simulink model "system_control"  (R2025b)
settings: Solver=VariableStepAuto  StartTime=0.0  StopTime=1  RelTol=1e-3
values from neighbouring files (symbols this model uses):
  adc_gain = (lim_adc(2)+1)/lim_voltage(2)    [sys_control.m]
  c1 = polyfit(lim_angles, lim_voltage, 1)    [sys_control.m]
  c2 = polyfit(lim_adc, lim_robot_speed, 1)    [sys_control.m]
  c3 = polyfit(lim_adc, lim_robot_angular_velocity, 1)    [sys_control.m]
  c4 = polyfit([0, lim_motor_speed(2)], lim_pwm, 1)    [sys_control.m]
  den_motor_tf = [J*La, J*Ra+b*La, b*Ra+Kt^2]    [sys_control.m]
  forward_kinematics = [ ... (first row only)    [sys_control.m]
  gear_ratio = 1/190    (= 0.00526315789474)    [sys_control.m]
  inverse_kinematics = [ ... (first row only)    [sys_control.m]
  lim_adc = [0, 2^bits-1]    [sys_control.m]
  lim_pwm = [0, 1]    [sys_control.m]
  lim_robot_angular_velocity = [-kinematic_resp(2), kinematic_resp(2)]    [sys_control.m]
  lim_robot_speed = [-kinematic_resp(1), kinematic_resp(1)]    [sys_control.m]
  lim_voltage = [0, 5]    [sys_control.m]
  noise_bias = 0    [sys_control.m]
  noise_bias_2 = 0    [sys_control.m]
  noise_frequency = 1000    [sys_control.m]
  noise_frequency_2 = 10000    [sys_control.m]
  noise_gain = 0.001    [sys_control.m]
  noise_gain_2 = 0.01    [sys_control.m]
  num_motor_tf = Kt    (= 0.076)    [sys_control.m]
  R = 0.3    [sys_control.m]
  vin = 24    [sys_control.m]
libraries: dspstat3 x2, simulink x2, dspfdesign x2, simulink_extras x1

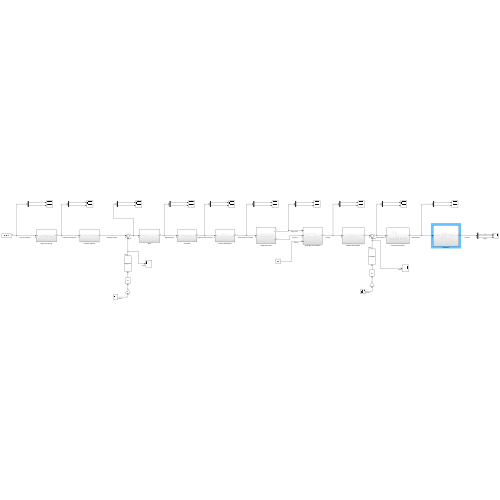
[thumbnail: Simulink's stored preview of the top-level diagram]
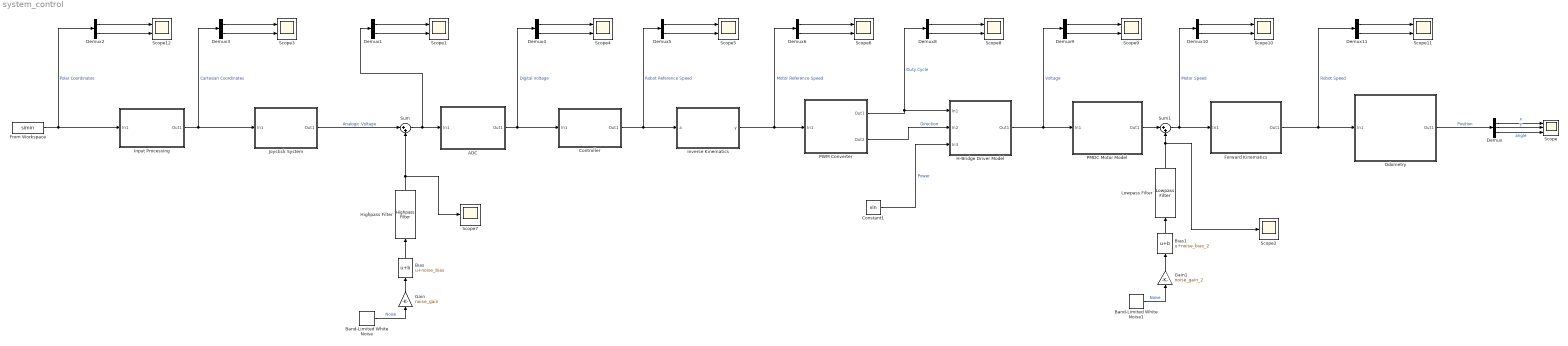
== system system_control ==
  ADC : Subsystem
  Band-Limited White Noise : simulink/Sources/Band-Limited White Noise  Cov=noise_power  Ts=1/noise_frequency  seed=[23341]
  Band-Limited White Noise1 : simulink/Sources/Band-Limited White Noise  Cov=noise_power_2  Ts=1/noise_frequency_2  seed=[23341]
  Bias : Bias  Bias=noise_bias  SaturateOnIntegerOverflow=off
  Bias1 : Bias  Bias=noise_bias_2  SaturateOnIntegerOverflow=off
  Constant1 : Constant  Value=vin
  Controller : Subsystem
  Demux : Demux  Outputs=3
  Demux{1..6,8..11} (10 alike) : Demux  Outputs=2
  Forward Kinematics : Subsystem
  From Workspace : FromWorkspace  VariableName=simin  OutputAfterFinalValue=Holding final value
  Gain : Gain  Gain=noise_gain
  Gain1 : Gain  Gain=noise_gain_2
  H-Bridge Driver Model : Subsystem
  Highpass Filter : dspfdesign/Highpass Filter  FilterType=FIR  DesignForMinimumOrder=on  FilterOrder=50  StopbandFrequency=10  PassbandFrequency=400  StopbandAttenuation=80  PassbandRipple=0.1  SampleRateMode=Specify on dialog  SampleRate=10000  SimulateUsing=Interpreted execution  roundingMode=Floor  coeffsDataTypeStr=fixdt(1,16)
  Input Processing : Subsystem
  Inverse Kinematics : Subsystem
  Joystick System : Subsystem
  Lowpass Filter : dspfdesign/Lowpass Filter  FilterType=FIR  DesignForMinimumOrder=on  FilterOrder=50  PassbandFrequency=8  StopbandFrequency=15  PassbandRipple=0.1  StopbandAttenuation=80  SampleRateMode=Specify on dialog  SampleRate=1000  SimulateUsing=Interpreted execution  roundingMode=Floor  coeffsDataTypeStr=fixdt(1,16)
  Odometry : Subsystem
  PMDC Motor Model : Subsystem
  PWM Converter : Subsystem
  Scope : Scope  NumInputPorts=3
      settings: ActiveDisplayYMinimum=-0.038312008816217151  ActiveDisplayYMaximum=0.34315381688886831  DataLoggingVariableName=odometry  DataLoggingSaveFormat=Structure
  Scope{1,3..6,8..12} (10 alike) : Scope  NumInputPorts=2
      Scope1 settings: ActiveDisplayYMinimum=1.060489809937327  ActiveDisplayYMaximum=5.7930389193730329  DataLoggingVariableName=joystick_analogic_voltage  DataLoggingSaveFormat=Structure
      Scope10 settings: ActiveDisplayYMinimum=-0.22999768707174573  ActiveDisplayYMaximum=0.57575148791845487  DataLoggingVariableName=motor_speed_rbv  DataLoggingSaveFormat=Structure
      Scope11 settings: ActiveDisplayYMinimum=-0.016441629327696137  ActiveDisplayYMaximum=0.1239488307824286  DataLoggingVariableName=robot_speed_rbv  DataLoggingSaveFormat=Structure
      Scope12 settings: ActiveDisplayYMinimum=-0.4195243112740431  ActiveDisplayYMaximum=1.1577249234748936  DataLoggingVariableName=input  DataLoggingSaveFormat=Structure
      Scope3 settings: ActiveDisplayYMinimum=-0.19779285643508393  ActiveDisplayYMaximum=1.1330880951594537  DataLoggingVariableName=joystick_inp  DataLoggingSaveFormat=Structure
      Scope4 settings: ActiveDisplayYMinimum=11.349880751221576  ActiveDisplayYMaximum=1081.1380282237869  DataLoggingVariableName=adc  DataLoggingSaveFormat=Structure
      Scope5 settings: ActiveDisplayYMinimum=0.074969930142674279  ActiveDisplayYMaximum=0.0752153728208186  DataLoggingVariableName=robot_speed_reference  DataLoggingSaveFormat=Structure
      Scope6 settings: ActiveDisplayYMinimum=-0.86358361035381748  ActiveDisplayYMaximum=0.54521612594059543  DataLoggingVariableName=motor_speed_reference  DataLoggingSaveFormat=Structure
      Scope8 settings: ActiveDisplayYMinimum=-0.12499999999999997  ActiveDisplayYMaximum=1.125  DataLoggingVariableName=pwm_duty_cycle  DataLoggingSaveFormat=Structure
      Scope9 settings: ActiveDisplayYMinimum=-29.510263929618766  ActiveDisplayYMaximum=25.592375366568909  DataLoggingVariableName=h_bridge_voltage  DataLoggingSaveFormat=Structure
  Scope2 : Scope
      settings: ActiveDisplayYMinimum=-0.30863024342846962  ActiveDisplayYMaximum=0.11012899050092259  DataLoggingVariableName=motor_speed_rbv1  DataLoggingSaveFormat=Structure
  Scope7 : Scope
      settings: ActiveDisplayYMinimum=-0.92976317089904748  ActiveDisplayYMaximum=0.28796558033489961  DataLoggingVariableName=motor_speed_rbv2  DataLoggingSaveFormat=Structure
  Sum : Sum  Inputs=|++
  Sum1 : Sum  Inputs=|++
  wires:
  Controller/1(Out1) -> Demux5/1, Inverse Kinematics/1(a)  "Robot Reference Speed"
  Inverse Kinematics/1(y) -> Demux6/1, PWM Converter/1(In1)  "Motor Reference Speed"
  PWM Converter/1(Out1) -> H-Bridge Driver Model/1(In1), Demux8/1  "Duty Cycle"
  H-Bridge Driver Model/1(Out1) -> Demux9/1, PMDC Motor Model/1(In1)  "Voltage"
  PMDC Motor Model/1(Out1) -> Sum1/1
  Demux1/2 -> Scope1/2
  Joystick System/1(Out1) -> Sum/1  "Analogic Voltage"
  Demux1/1 -> Scope1/1
  Sum/1 -> Demux1/1, ADC/1(In1)
  Band-Limited White Noise/1 -> Gain/1  "Noise"
  Bias/1 -> Highpass Filter/1
  Gain/1 -> Bias/1
  Demux3/1 -> Scope3/1
  Demux3/2 -> Scope3/2
  ADC/1(Out1) -> Demux4/1, Controller/1(In1)  "Digital Voltage"
  Demux4/1 -> Scope4/1
  Demux4/2 -> Scope4/2
  Demux5/1 -> Scope5/1
  Demux5/2 -> Scope5/2
  Demux6/1 -> Scope6/1
  Demux6/2 -> Scope6/2
  Demux8/2 -> Scope8/2
  Demux8/1 -> Scope8/1
  PWM Converter/2(Out2) -> H-Bridge Driver Model/2(In2)  "Direction"
  Constant1/1 -> H-Bridge Driver Model/3(In3)  "Power"
  Demux9/2 -> Scope9/2
  Demux9/1 -> Scope9/1
  Demux10/1 -> Scope10/1
  Demux10/2 -> Scope10/2
  Forward Kinematics/1(Out1) -> Demux11/1, Odometry/1(In1)  "Robot Speed"
  Demux11/2 -> Scope11/2
  Demux11/1 -> Scope11/1
  Odometry/1(Out1) -> Demux/1  "Position"
  Demux/1 -> Scope/1  "x"
  Demux/2 -> Scope/2  "y"
  Demux/3 -> Scope/3  "angle"
  Band-Limited White Noise1/1 -> Gain1/1  "Noise"
  Gain1/1 -> Bias1/1
  Sum1/1 -> Demux10/1, Forward Kinematics/1(In1)  "Motor Speed"
  Bias1/1 -> Lowpass Filter/1
  Lowpass Filter/1 -> Scope2/1, Sum1/2
  Highpass Filter/1 -> Sum/2, Scope7/1
  Input Processing/1(Out1) -> Demux3/1, Joystick System/1(In1)  "Cartesian Coordinates"
  From Workspace/1 -> Demux2/1, Input Processing/1(In1)  "Polar Coordinates"
  Demux2/1 -> Scope12/1
  Demux2/2 -> Scope12/2

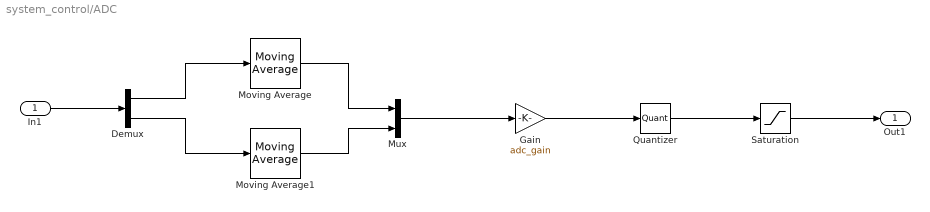
== system system_control/ADC ==
  In1 : Inport
  Demux : Demux  Outputs=2
  Gain : Gain  Gain=adc_gain
  Moving Average : dspstat3/Moving Average  Method=Sliding window  ForgettingFactorPort=off  SpecifyWindowLength=on  WindowLength=4  OverlapLength=3  AllowArbitraryInputLength=off  ForgettingFactor=0.9  SimulateUsing=Interpreted execution
  Moving Average1 : dspstat3/Moving Average  Method=Sliding window  ForgettingFactorPort=off  SpecifyWindowLength=on  WindowLength=4  OverlapLength=3  AllowArbitraryInputLength=off  ForgettingFactor=0.9  SimulateUsing=Interpreted execution
  Mux : Mux  Inputs=2
  Quantizer : Quantizer
  Saturation : Saturate  UpperLimit=lim_adc(2)  LowerLimit=lim_adc(1)  ZeroCross=off
  Out1 : Outport
  wires:
  Gain/1 -> Quantizer/1
  Quantizer/1 -> Saturation/1
  Saturation/1 -> Out1/1
  In1/1 -> Demux/1
  Demux/1 -> Moving Average/1
  Mux/1 -> Gain/1
  Moving Average/1 -> Mux/1
  Moving Average1/1 -> Mux/2
  Demux/2 -> Moving Average1/1

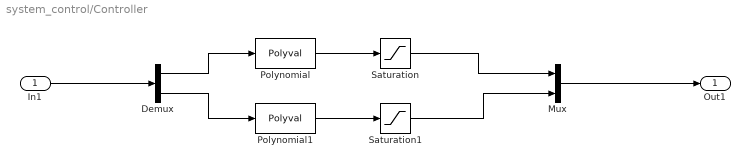
== system system_control/Controller ==
  In1 : Inport
  Demux : Demux  Outputs=2
  Mux : Mux  Inputs=2
  Polynomial : Polyval  Coefs=c2
  Polynomial1 : Polyval  Coefs=c3
  Saturation : Saturate  UpperLimit=lim_robot_speed(2)  LowerLimit=lim_robot_speed(1)
  Saturation1 : Saturate  UpperLimit=lim_robot_angular_velocity(2)  LowerLimit=lim_robot_angular_velocity(1)
  Out1 : Outport
  wires:
  Demux/1 -> Polynomial/1
  Demux/2 -> Polynomial1/1
  Polynomial/1 -> Saturation/1
  Saturation/1 -> Mux/1
  Polynomial1/1 -> Saturation1/1
  Saturation1/1 -> Mux/2
  Mux/1 -> Out1/1
  In1/1 -> Demux/1

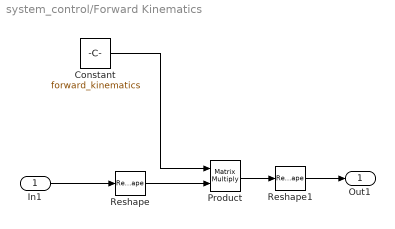
== system system_control/Forward Kinematics ==
  In1 : Inport
  Constant : Constant  Value=forward_kinematics
  Product : Product  Multiplication=Matrix(*)
  Reshape : Reshape  OutputDimensionality=Column vector (2-D)
  Reshape1 : Reshape
  Out1 : Outport
  wires:
  Product/1 -> Reshape1/1
  In1/1 -> Reshape/1
  Constant/1 -> Product/1
  Reshape/1 -> Product/2
  Reshape1/1 -> Out1/1

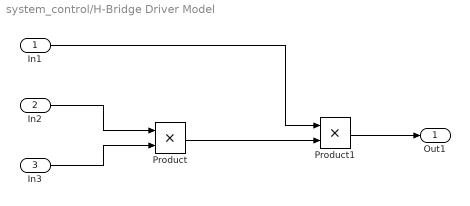
== system system_control/H-Bridge Driver Model ==
  In1 : Inport
  In2 : Inport  Port=2
  In3 : Inport  Port=3
  Product : Product
  Product1 : Product
  Out1 : Outport
  wires:
  In2/1 -> Product/1
  In3/1 -> Product/2
  In1/1 -> Product1/1
  Product/1 -> Product1/2
  Product1/1 -> Out1/1

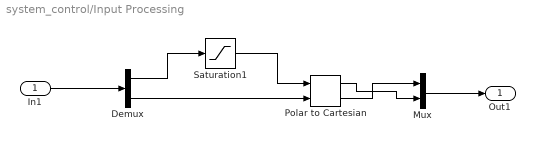
== system system_control/Input Processing ==
  In1 : Inport
  Demux : Demux  Outputs=2
  Mux : Mux  Inputs=2
  Polar to Cartesian : simulink_extras/Transformations/Polar to Cartesian
  Saturation1 : Saturate  UpperLimit=1  LowerLimit=0
  Out1 : Outport
  wires:
  In1/1 -> Demux/1
  Demux/1 -> Saturation1/1
  Demux/2 -> Polar to Cartesian/2
  Saturation1/1 -> Polar to Cartesian/1
  Polar to Cartesian/2 -> Mux/1
  Mux/1 -> Out1/1
  Polar to Cartesian/1 -> Mux/2

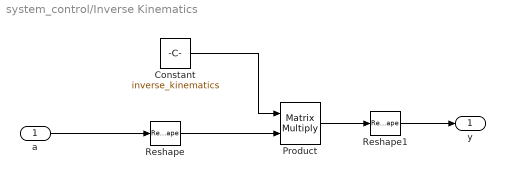
== system system_control/Inverse Kinematics ==
  a : Inport
  Constant : Constant  Value=inverse_kinematics
  Product : Product  Multiplication=Matrix(*)
  Reshape : Reshape  OutputDimensionality=Column vector (2-D)
  Reshape1 : Reshape
  y : Outport
  wires:
  Constant/1 -> Product/1
  Product/1 -> Reshape1/1
  a/1 -> Reshape/1
  Reshape/1 -> Product/2
  Reshape1/1 -> y/1

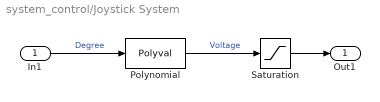
== system system_control/Joystick System ==
  In1 : Inport
  Polynomial : Polyval  Coefs=c1
  Saturation : Saturate  UpperLimit=lim_voltage(2)  LowerLimit=lim_voltage(1)  ZeroCross=off
  Out1 : Outport
  wires:
  Polynomial/1 -> Saturation/1  "Voltage"
  In1/1 -> Polynomial/1  "Degree"
  Saturation/1 -> Out1/1

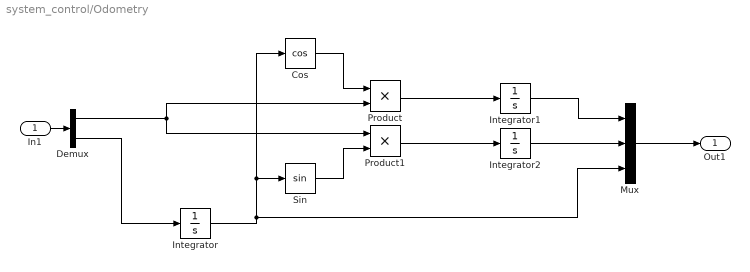
== system system_control/Odometry ==
  In1 : Inport
  Cos : Trigonometry  Operator=cos
  Demux : Demux  Outputs=2
  Integrator : Integrator
  Integrator1 : Integrator
  Integrator2 : Integrator
  Mux : Mux  Inputs=3
  Product : Product
  Product1 : Product
  Sin : Trigonometry
  Out1 : Outport
  wires:
  Integrator/1 -> Mux/3, Cos/1, Sin/1
  Demux/2 -> Integrator/1
  In1/1 -> Demux/1
  Cos/1 -> Product/1
  Demux/1 -> Product1/1, Product/2
  Sin/1 -> Product1/2
  Product/1 -> Integrator1/1
  Product1/1 -> Integrator2/1
  Integrator2/1 -> Mux/2
  Integrator1/1 -> Mux/1
  Mux/1 -> Out1/1

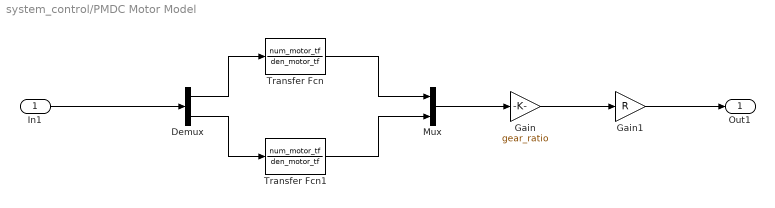
== system system_control/PMDC Motor Model ==
  In1 : Inport
  Demux : Demux  Outputs=2
  Gain : Gain  Gain=gear_ratio
  Gain1 : Gain  Gain=R
  Mux : Mux  Inputs=2
  Transfer Fcn : TransferFcn  Numerator=num_motor_tf  Denominator=den_motor_tf
  Transfer Fcn1 : TransferFcn  Numerator=num_motor_tf  Denominator=den_motor_tf
  Out1 : Outport
  wires:
  In1/1 -> Demux/1
  Gain/1 -> Gain1/1
  Demux/1 -> Transfer Fcn/1
  Demux/2 -> Transfer Fcn1/1
  Transfer Fcn/1 -> Mux/1
  Transfer Fcn1/1 -> Mux/2
  Mux/1 -> Gain/1
  Gain1/1 -> Out1/1

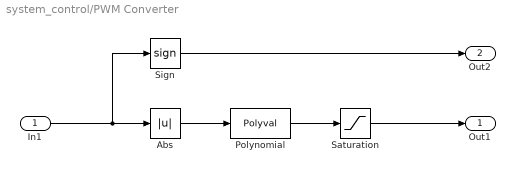
== system system_control/PWM Converter ==
  In1 : Inport
  Abs : Abs  ZeroCross=off  SaturateOnIntegerOverflow=off
  Polynomial : Polyval  Coefs=c4
  Saturation : Saturate  UpperLimit=lim_pwm(2)  LowerLimit=lim_pwm(1)  ZeroCross=off
  Sign : Signum  ZeroCross=off
  Out1 : Outport
  Out2 : Outport  Port=2
  wires:
  In1/1 -> Sign/1, Abs/1
  Polynomial/1 -> Saturation/1
  Saturation/1 -> Out1/1
  Abs/1 -> Polynomial/1
  Sign/1 -> Out2/1
